simulink model "gm_AGC"  (R2021a)
settings: Solver=FixedStepAuto  StartTime=0.0  StopTime=400  RelTol=1e-3  EnableMultiTasking=on
model workspace (MAT data in the model file):
  th = 0
libraries: dspsrcs4 x2, hdlsllib x1
settings Model: EnablePacing=on  Creator=guido  LastModifiedBy=guido
settings DataIOCC: ExternalInput=x_ts
settings OptimizationCC: BlockReduction=off  ConditionallyExecuteInputs=off
settings DebuggingCC: SignalRangeChecking=warning  InheritedTsInSrcMsg=none  SingleTaskRateTransMsg=error

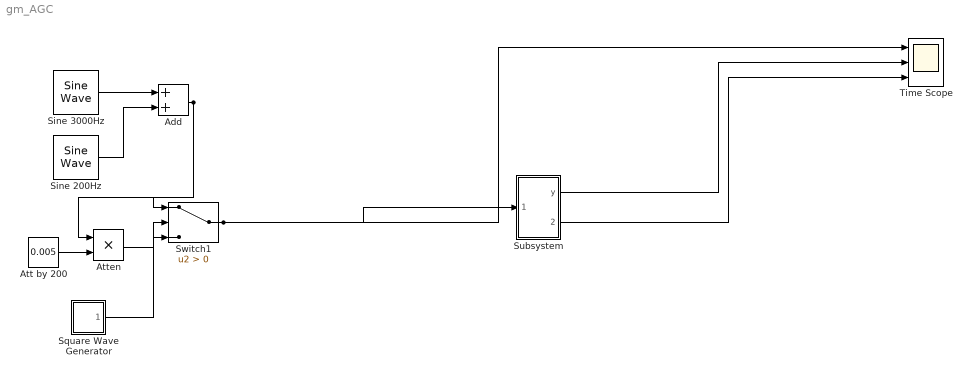
== system gm_AGC ==
  Add : Sum  AccumDataTypeStr=int32  OutDataTypeStr=int32
  Att by 200 : Constant  Value=0.005
  Atten : Product  OutDataTypeStr=int16
  Sine 200Hz : dspsrcs4/Sine Wave  Amplitude=16384  Frequency=200  Phase=0  SampleMode=Discrete  OutComplex=Real  CompMethod=Table lookup  TableSize=Speed  SampleTime=1/48000  SamplesPerFrame=1  ResetState=Restart at time zero  OutputFrames=off  dataType=Fixed-point  wordLen=16  udDataType=sfix(16)  fracBitsMode=Best precision  numFracBits=14  OutDataTypeStr=fixdt(1,16)  LastOutDataTypeStr=fixdt(1,16)
  Sine 3000Hz : dspsrcs4/Sine Wave  Amplitude=16384  Frequency=3000  Phase=0  SampleMode=Discrete  OutComplex=Real  CompMethod=Table lookup  TableSize=Speed  SampleTime=1/48000  SamplesPerFrame=1  ResetState=Restart at time zero  OutputFrames=off  dataType=Fixed-point  wordLen=16  udDataType=sfix(16)  fracBitsMode=Best precision  numFracBits=0  OutDataTypeStr=fixdt(1,16)  LastOutDataTypeStr=fixdt(1,16)
  Square Wave Generator : Subsystem  Tag=DecoupledSystem
  Subsystem : Subsystem
  Switch1 : Switch  Criteria=u2 > Threshold
  Time Scope : Scope  NumInputPorts=3
  wires:
  Subsystem/2(Out2) -> Time Scope/3
  Subsystem/1(y) -> Time Scope/2
  Add/1 -> Atten/1, Switch1/1
  Square Wave Generator/1(Out1) -> Switch1/2
  Att by 200/1 -> Atten/2
  Atten/1 -> Switch1/3
  Sine 200Hz/1 -> Add/2
  Sine 3000Hz/1 -> Add/1
  Switch1/1 -> Subsystem/1(In1), Time Scope/1

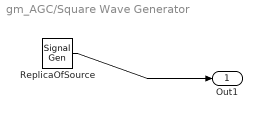
== system gm_AGC/Square Wave Generator ==
  ReplicaOfSource : SignalGenerator  WaveForm=square  Amplitude=256  Frequency=0.5
  Out1 : Outport  LockScale=on
  wires:
  ReplicaOfSource/1 -> Out1/1

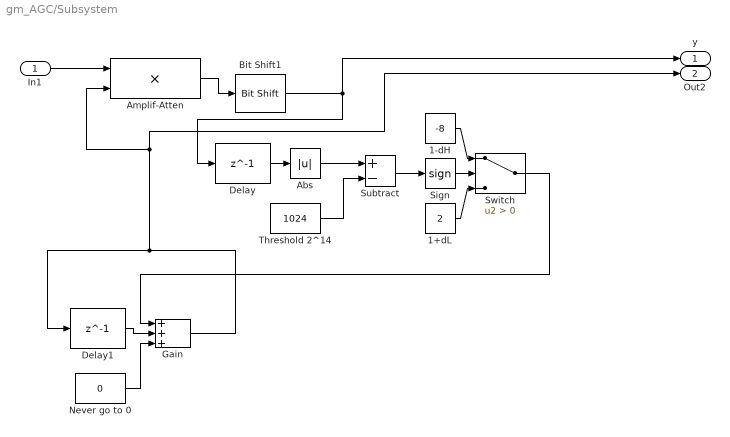
== system gm_AGC/Subsystem ==
  In1 : Inport
  1+dL : Constant  Value=2  OutDataTypeStr=int16
  1-dH : Constant  Value=-8  OutDataTypeStr=int16
  Abs : Abs  OutDataTypeStr=int32  SaturateOnIntegerOverflow=on
  Amplif-Atten : Product  OutDataTypeStr=fixdt(1,22,0)  SaturateOnIntegerOverflow=on
  Bit Shift1 : hdlsllib/Logic and Bit Operations/Bit Shift  mode=Shift Right Arithmetic  N=10
  Delay : Delay  DelayLength=1  InitialCondition=0  UseCircularBuffer=on
  Delay1 : Delay  DelayLength=1  InitialCondition=1  UseCircularBuffer=on
  Gain : Sum  Inputs=+++  OutDataTypeStr=fixdt(0,14,0)  SaturateOnIntegerOverflow=on
  Never go to 0 : Constant  Value=0  OutDataTypeStr=int16
  Sign : Signum
  Subtract : Sum  Inputs=+-  AccumDataTypeStr=int32  OutDataTypeStr=int32  SaturateOnIntegerOverflow=on
  Switch : Switch  Criteria=u2 > Threshold  OutDataTypeStr=int8  SaturateOnIntegerOverflow=on
  Threshold 2^14 : Constant  Value=1024  OutDataTypeStr=int32
  y : Outport
  Out2 : Outport  Port=2
  wires:
  In1/1 -> Amplif-Atten/1
  Never go to 0/1 -> Gain/3
  Bit Shift1/1 -> Delay/1, y/1
  Delay1/1 -> Gain/2
  Threshold 2^14/1 -> Subtract/2
  1-dH/1 -> Switch/1
  Amplif-Atten/1 -> Bit Shift1/1
  Subtract/1 -> Sign/1
  1+dL/1 -> Switch/3
  Sign/1 -> Switch/2
  Abs/1 -> Subtract/1
  Switch/1 -> Gain/1
  Gain/1 -> Delay1/1, Amplif-Atten/2, Out2/1
  Delay/1 -> Abs/1
